simulink model "comm_test"  (R2014a)
settings: Solver=ode4  StartTime=0.0  StopTime=inf  FixedStep=0.001  RelTol=1e-3
libraries: simulink x1, SimulinkExecutionControl x1
settings Model: Creator=Tulga Ersal  LastModifiedBy=zhengys
settings OptimizationCC: ExpressionDepthLimit=2147483647
settings DebuggingCC: UnderspecifiedInitializationDetection=Classic  StateNameClashWarn=warning

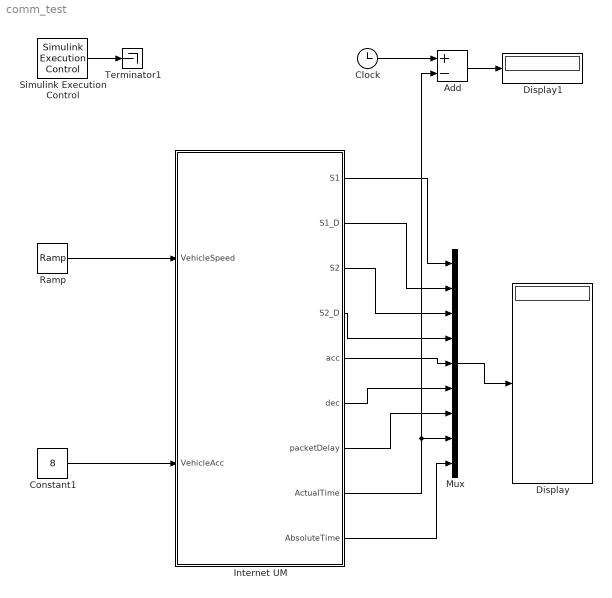
== system comm_test ==
  Add : Sum  Inputs=+-
  Clock : Clock
  Constant1 : Constant  Value=8
  Display : Display
  Display1 : Display
  Internet UM : Subsystem
  Mux : Mux  Inputs=9
  Ramp : simulink/Sources/Ramp  slope=1  start=0  X0=0
  Simulink Execution Control : SimulinkExecutionControl/Simulink Execution Control  proc_pri=REALTIME_PRIORITY_CLASS  thread_pri=THREAD_PRIORITY_TIME_CRITICAL  rt_sim=on  factor=1  ovrrun=Continue execution  Ts=4e-3
  Terminator1 : Terminator
  wires:
  Simulink Execution Control/1 -> Terminator1/1
  Mux/1 -> Display/1
  Ramp/1 -> Internet UM/1(VehicleSpeed)
  Constant1/1 -> Internet UM/2(VehicleAcc)
  Internet UM/5(acc) -> Mux/5
  Internet UM/4(S2_D) -> Mux/4
  Internet UM/6(dec) -> Mux/6
  Internet UM/3(S2) -> Mux/3
  Internet UM/7(packetDelay) -> Mux/7
  Internet UM/2(S1_D) -> Mux/2
  Internet UM/8(ActualTime) -> Add/2, Mux/8
  Internet UM/1(S1) -> Mux/1
  Internet UM/9(AbsoluteTime) -> Mux/9
  Clock/1 -> Add/1
  Add/1 -> Display1/1

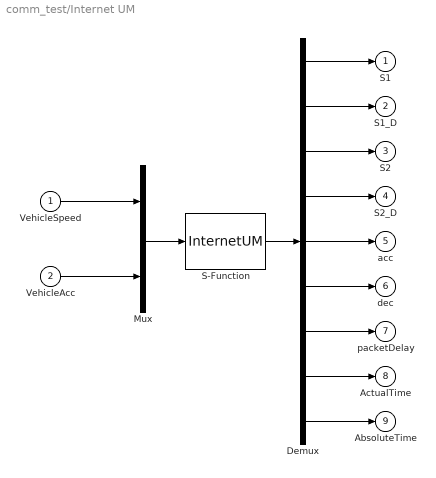
== system comm_test/Internet UM ==
  VehicleSpeed : Inport
  VehicleAcc : Inport  Port=2
  Demux : Demux  Outputs=9
  Mux : Mux  Inputs=2
  S-Function : S-Function  FunctionName=InternetUM  EnableBusSupport=off
  S1 : Outport
  S1_D : Outport  Port=2
  S2 : Outport  Port=3
  S2_D : Outport  Port=4
  acc : Outport  Port=5
  dec : Outport  Port=6
  packetDelay : Outport  Port=7
  ActualTime : Outport  Port=8
  AbsoluteTime : Outport  Port=9
  wires:
  VehicleSpeed/1 -> Mux/1
  Demux/1 -> S1/1
  Demux/2 -> S1_D/1
  Mux/1 -> S-Function/1
  S-Function/1 -> Demux/1
  VehicleAcc/1 -> Mux/2
  Demux/3 -> S2/1
  Demux/4 -> S2_D/1
  Demux/5 -> acc/1
  Demux/6 -> dec/1
  Demux/7 -> packetDelay/1
  Demux/8 -> ActualTime/1
  Demux/9 -> AbsoluteTime/1
